simulink model "design_project_openloop_linear_bk_3"  (R2023b)
settings: Solver=VariableStepAuto  StartTime=0.0  StopTime=500  RelTol=1e-3
settings Model: Creator=18265  LastModifiedBy=qingyu
settings SolverCC: AlgebraicLoopSolver=TrustRegion
settings DataIOCC: ReturnWorkspaceOutputs=off
settings DebuggingCC: UnconnectedInputMsg=warning  UnconnectedOutputMsg=warning  UnconnectedLineMsg=warning  ArithmeticOperatorsInVariantConditions=warning
settings ModelReferenceCC: EnableRefExpFcnMdlSchedulingChecks=on
settings SFSimCC: CustomCodeUndefinedFunction=UseInterfaceOnly

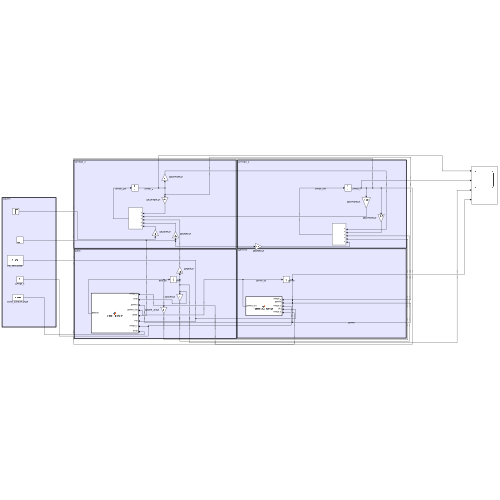
[thumbnail: Simulink's stored preview of the top-level diagram]
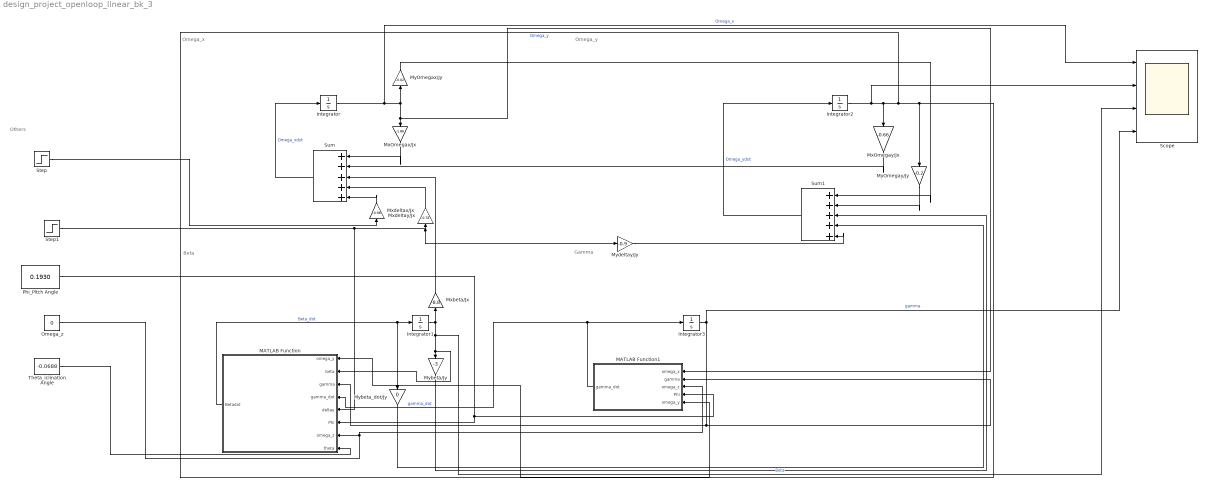
== system design_project_openloop_linear_bk_3 ==
  note: Others
  note: Gamma
  note: Beta
  note: Omega_y
  note: Omega_x
  Integrator : Integrator  InitialCondition=0.1
  Integrator1 : Integrator  InitialCondition=0.05
  Integrator2 : Integrator  InitialCondition=0.1
  Integrator3 : Integrator  InitialCondition=0.05
  MATLAB Function : MATLAB Function  TreatAsAtomicUnit=on
  MATLAB Function1 : MATLAB Function  TreatAsAtomicUnit=on
  MxOmegax/Jx : Gain  Gain=-1.86
  MxOmegay/Jx : Gain  Gain=-0.66
  Mxbeta/Jx : Gain  Gain=-8.8
  Mxdeltax/Jx : Gain  Gain=-0.98
  Mxdeltay/Jx : Gain  Gain=-0.78
  MyOmegax/Jy : Gain  Gain=-0.02
  MyOmegay/Jy : Gain  Gain=-0.2
  Mybeta/Jy : Gain  Gain=-3
  Mybeta_dot/Jy : Gain  Gain=0
  Mydeltay/Jy : Gain  Gain=-0.9
  Omega_z : Constant  Value=0
  Phi_Pitch Angle : Constant  Value=0.1930
  Scope : Scope  NumInputPorts=4
  Step : Step  After=0  SampleTime=0
  Step1 : Step  After=0  SampleTime=0
  Sum : Sum  Inputs=|+++++
  Sum1 : Sum  Inputs=|+++++
  Theta_iclination Angle : Constant  Value=-0.0688
  wires:
  Sum/1 -> Integrator/1  "Omega_xdot"
  Integrator/1 -> Scope/1, MATLAB Function1/1(omega_x), MxOmegax/Jx/1, MyOmegax/Jy/1  "Omega_x"
  MATLAB Function/1(Betadot) -> Integrator1/1, Mybeta_dot/Jy/1  "Beta_dot"
  Integrator1/1 -> Mxbeta/Jx/1, Scope/3, MATLAB Function/2(beta), Mybeta/Jy/1  "Beta"
  Sum1/1 -> Integrator2/1  "Omega_ydot"
  Integrator2/1 -> Scope/2, MATLAB Function1/5(omega_y), MATLAB Function/1(omega_y), MyOmegay/Jy/1, MxOmegay/Jx/1  "Omega_y"
  MATLAB Function1/1(gamma_dot) -> Integrator3/1, MATLAB Function/4(gamma_dot)  "gamma_dot"
  Integrator3/1 -> MATLAB Function1/2(gamma), MATLAB Function/3(gamma), Scope/4  "gamma"
  MxOmegax/Jx/1 -> Sum/1
  MxOmegay/Jx/1 -> Sum/2
  Mxbeta/Jx/1 -> Sum/3
  Step/1 -> Mxdeltax/Jx/1
  Step1/1 -> MATLAB Function/5(deltay), Mydeltay/Jy/1, Mxdeltay/Jx/1
  Mxdeltay/Jx/1 -> Sum/4
  Mxdeltax/Jx/1 -> Sum/5
  MyOmegax/Jy/1 -> Sum1/1
  MyOmegay/Jy/1 -> Sum1/2
  Mybeta/Jy/1 -> Sum1/3
  Mybeta_dot/Jy/1 -> Sum1/4
  Mydeltay/Jy/1 -> Sum1/5
  Phi_Pitch Angle/1 -> MATLAB Function1/4(Phi), MATLAB Function/6(Phi)
  Omega_z/1 -> MATLAB Function1/3(omega_z), MATLAB Function/7(omega_z)
  Theta_iclination Angle/1 -> MATLAB Function/8(theta)

== matlab function design_project_openloop_linear_bk_3/MATLAB Function1 ==
  data: omega_x input; gamma_dot output; gamma input; omega_z input; Phi input; omega_y input
function gamma_dot = gammadot_transfer(omega_x,gamma,omega_z,Phi,omega_y)

gamma_dot = 0;
gamma_dot = gamma_dot + omega_x;
gamma_dot = gamma_dot - tand(Phi)*omega_y;

== matlab function design_project_openloop_linear_bk_3/MATLAB Function ==
  data: omega_y input; Betadot output; beta input; gamma input; gamma_dot input; deltay input; Phi input; omega_z input; theta input
function Betadot = Betadot_transfer(omega_y,beta,gamma,gamma_dot,deltay,Phi,omega_z,theta)

g = 9.81;%Gravitational Acceleration
v = 350.3552;%velocity
alpha = Phi - theta;
Z_deltay = -2018.0457;%Partial Z / Partial deltay
m = 320;%mass
P = 20000;%thrust
Z_beta = 13273.1810;

Betadot = 0;
Betadot = Betadot + cosd(theta)/cosd(Phi)*omega_y;
Betadot = Betadot - (P-Z_beta)/(m*v)*beta;
Betadot = Betadot + (g/v)*sind(theta)*beta;
Betadot = Betadot + (g/v)*cosd(Phi)*gamma;
Betadot = Betadot + alpha*gamma_dot;
Betadot = Betadot + Z_deltay/(m*v)*deltay;
